simulink model "Copy_of_finalMG"  (R2025b)
settings: Solver=FixedStepAuto  StartTime=0.0  StopTime=.072  FixedStep=Ts  MaxStep=1e-4  RelTol=1e-3  EnableMultiTasking=on
PreLoadFcn:
  | Ts = 1e-5;
  | fsw = 1e3;
undefined symbols (not defined in the file or in its folder): localhost
libraries: nesl_utility x27, ee_lib x16, fl_lib x10, modbuslib x5, simulink x2, batteryecm_lib x1, eePwmGeneratorTwoLevel x1
CloseFcn:
  | try,close(h1_TwoLevelPWMGenerator),end
  | clear h1_TwoLevelPWMGenerator tout
  | 
  | clear simlog_TwoLevelPWMGenerator
  | clear logsout_TwoLevelPWMGenerator
  | clear Ts fsw
Description:
  | Three-Phase Two-Level PWM Generator
settings Model: Creator=The MathWorks, Inc.  LastModifiedBy=mattpenne
settings SolverCC: AlgebraicLoopSolver=TrustRegion  MaxZcPerStep=1.0
settings DataIOCC: LimitDataPoints=on  MaxDataPoints=50000  SaveFormat=Array  SaveOutput=off  SignalLogging=off  DSMLogging=off  SaveTime=off  ReturnWorkspaceOutputs=off  SignalLoggingName=logsout_TwoLevelPWMGenerator
settings OptimizationCC: ReuseModelBlockBuffer=off  LifeSpan=inf
settings DebuggingCC: AlgebraicLoopMsg=error  SolverPrmCheckMsg=warning  MultiTaskRateTransMsg=warning  UnconnectedInputMsg=warning  UnconnectedOutputMsg=warning  UnconnectedLineMsg=warning  AllowSymbolicDim=off  SFUnexpectedBacktrackingDiag=warning  SFNoUnconditionalDefaultTransitionDiag=warning  SFExecutionAtInitializationDiag=none  ArithmeticOperatorsInVariantConditions=warning
settings HardwareCC: ProdBitPerPointer=32.0  ProdBitPerSizeT=32.0  ProdBitPerPtrDiffT=32.0  ProdLargestAtomicFloat=None  ProdIntDivRoundTo=Undefined  ProdEndianess=Unspecified  ProdWordSize=32.0  ProdHWDeviceType=32-bit Generic
settings ModelReferenceCC: EnableRefExpFcnMdlSchedulingChecks=on  PropagateSignalLabelsOutOfModel=off
settings SFSimCC: SimUseLocalCustomCode=off  CustomCodeUndefinedFunction=UseInterfaceOnly
settings RTWCC: RTWUseLocalCustomCode=off  GPUComputeCapability=3.5  DLArmComputeVersion=19.05
settings CodeAppCC: StateflowObjectComments=on
settings GRTTargetCC: TargetLangStandard=C89/C90 (ANSI)
settings ConfigComp: CovMetricSettings=dw  CovSaveCumulativeToWorkspaceVar=on  CovSaveSingleToWorkspaceVar=on  CovExternalEMLEnable=off  CovSFcnEnable=off
settings SimscapeCC: SimscapeLogType=all  SimscapeLogSimulationStatistics=on  SimscapeLogName=simlog_TwoLevelPWMGenerator  SimscapeLogDataHistory=50000.0

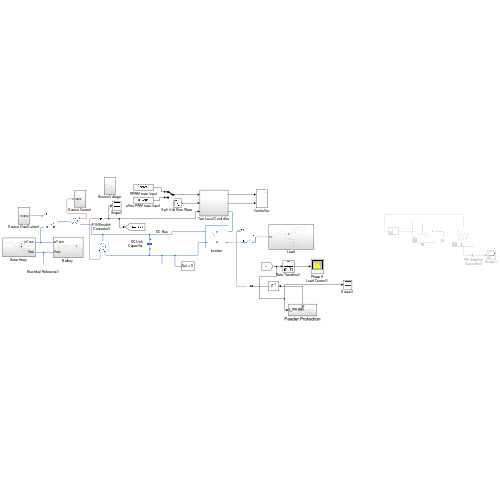
[thumbnail: Simulink's stored preview of the top-level diagram]
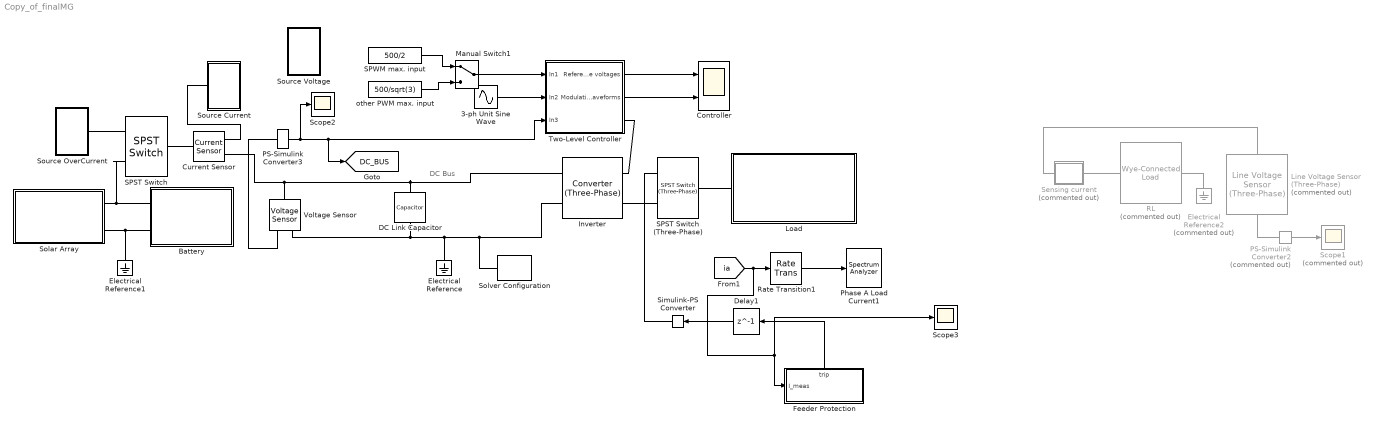
== system Copy_of_finalMG ==
  note: DC Bus
  3-ph Unit Sine Wave : Sin  Frequency=2*pi*60  Phase="[0  -2*pi/3  2*pi/3] + pi/2"  SampleTime=0
  Battery : Subsystem
  Controller : Scope  NumInputPorts=2
      settings: ActiveDisplayYMinimum=-250  ActiveDisplayYMaximum=250  DataLoggingVariableName=ScopeData2  DataLoggingSaveFormat=Array
  Current Sensor : fl_lib/Electrical/Electrical Sensors/Current Sensor
  DC Link Capacitor : ee_lib/Passive/Capacitor  cap_option=ee.enum.passive.capacitor.capOption.const  c=.001 F  Cvec=[1e-05, 1e-06] F  Vvec=[0, 10] V  CV_table_symmetry=ee.enum.passive.capacitor.tableSymmetry.yes  f_vec=[1, 10] kHz  DFext_vec=[.8, 1.2]  enable_C_tol=ee.enum.toleranceApplication.none  averaging_period=0 s  C_tol=5  tol_distribution=ee.enum.toleranceDistribution.uniform  nSigma=4  r=1e-6 Ohm  g=0 1/Ohm  enable_operating_limits=ee.enum.enable.no  operating_limit_action=ee.enum.passive.reportOpLim.warn  max_working_voltage_range=[-25, 25] V  power_rating=1 W  maxTemperature=85 degC  thermalEnable=false  thermalMass=1 J/K  i_specify=off  i_priority=None  i=0 A  i_nominal_specify=off  i_nominal_value=1  i_nominal_unit=A  v_specify=off  v_priority=None  v=0 V  v_nominal_specify=off  v_nominal_value=1  v_nominal_unit=V  vc_specify=off  vc_priority=High  vc=0 V  vc_nominal_specify=off  vc_nominal_value=1  vc_nominal_unit=V  T_specify=off  T_priority=None  T=298.15 K  T_nominal_specify=off  T_nominal_value=1  T_nominal_unit=K
  Delay1 : Delay  DelayLength=1  InitialCondition=0
  Electrical Reference : fl_lib/Electrical/Electrical Elements/Electrical Reference
  Electrical Reference1 : fl_lib/Electrical/Electrical Elements/Electrical Reference
  Electrical Reference2 : fl_lib/Electrical/Electrical Elements/Electrical Reference  Commented=on
  Feeder Protection : Subsystem
      settings: PortSchema="{\"entries\":[{\"content\":{\"sides\":[{\"content\":{\"connectorIds\":[\"In1\"]},\"type\":\"ConnectorPlacement.EquallySpacedRectSide\",\"uuid\":\"0697f356-98a9-46a1-9ee7-a2f5bd8a9ce9\"},{\"content\":{\"side\":\"RIGHT\"},\"type\":\"ConnectorPlacement.EquallySpacedRectSide\",\"uuid\":\"d4eac892-3d6d-4f1e-85a9-65422e23728d\"},{\"content\":{\"connectorIds\":[\"Out1\"],\"side\":\"TOP\"},\"type\":\"ConnectorPlacement.EquallySpacedRectSide\",\"uuid\":\"7d3e352e-ceac-4059-a935-aae4fffcf2cb\"}]},\"type\":\"ConnectorPlacement.EquallySpacedConnector\",\"uuid\":\"a2d9bf32-257e-4270-ae17-1068e4e35877\"}],\"packageUris\":[\"http://schema.mathworks.com/mf0/Connector/R2020b\"],\"version\":\"1.0\"}"
  Inverter : ee_lib/Semiconductors & Converters/Converters/Converter (Three-Phase)  port_option=ee.enum.threePhasePort.composite  fidelity_option=ee.enum.converters.fidelity.detailed  device_type=3  showThermalPort=false  K=0  Vth=0.5 V  Vgt=1 V  Vgt_off=-1 V  Ih=1 A  Vf=0.8 V  Ron=0.001 Ohm  Rds=0.001 Ohm  Goff=1e-5 1/Ohm  Eon_scalar=22.86e-3 J  Eoff_scalar=17.14e-3 J  Eoff_natural_commutation=10e-3 J  Voff=300 V  Iout_scalar=600 A  onCurrentMeasDelay=0 s  useCurrentFromPreviousCycle=false  useVoltageFromPreviousCycle=false  diode_param=2  diode_Vf=0.8 V  diode_Ron=0.001 Ohm  diode_Goff=1e-5 1/Ohm  diode_C=50 nF  diode_iRM=-235 A  diode_iF=300 A  diode_idot=-50 A/us  diode_trr_param=1  diode_trr_factor=3  diode_trr=15 us  diode_Qrr=1.5e+3 s*uA  diode_rec_loss_model=ee.enum.diode.reverseRecoveryModel.fixed  diode_ErecVal=0 J  diode_scaleWithIandV=false  diode_ErecMat=zeros(2, 3) J  diode_TjrecVec=[298.15, 398.15] K  diode_IfrecVec=[.1, 1, 10] A  diode_IrecVal=10 A  diode_VrecVal=10 V  diode_tFilter=1 / 1000 / 100 s  thermal_network_parameterization=ee.enum.thermalNetworkTopology.external  Rth=[.08, .5] K/W  Rth_Cauer=[.08, .1, .5] K/W  Rth_Foster=[.08, .14, .22, .16] K/W  thermal_mass_parameterization=ee.enum.thermalNetwork.timeconstant  thermal_mass=[.01, .5] J/K  thermal_mass_Cauer=[.01, .1, .5] J/K  thermal_mass_Foster=[.001, .005, .05, .5] J/K  thermal_time_constant=[.001, .2] s  thermal_time_constant_Cauer=[.001, .1, .2] s  thermal_time_constant_Foster=[7e-05, .0007, .01, .08] s  thermal_mass_initial_temperatures=[25, 25] degC  thermal_mass_initial_temperatures_Cauer=[25, 25, 25] degC  junction_thermal_mass=0.01 J/K  Tvec_initial_Foster=[25, 25, 25, 25] degC  snubber_type=0  Cs=1e-7 F  Rs=0.1 Ohm  Vce_loss=[0, 150, 300] V
  Line Voltage Sensor (Three-Phase) : ee_lib/Sensors & Transducers/Line Voltage Sensor (Three-Phase)  Commented=on
  Load : Subsystem
  Manual Switch1 : ManualSwitch
  PS-Simulink Converter2 : nesl_utility/PS-Simulink Converter  Commented=on  PhysicalDomain=network_engine_domain  SubClassName=ps_output  LeftPortType=input  RightPortType=output  PseudoPeriodic=off  Frequencies=[]  VectorFormat=inherit  Unit=inherit  AffineConversion=off
  PS-Simulink Converter3 : nesl_utility/PS-Simulink Converter  PhysicalDomain=network_engine_domain  SubClassName=ps_output  LeftPortType=input  RightPortType=output  PseudoPeriodic=off  Frequencies=[]  VectorFormat=inherit  Unit=inherit  AffineConversion=off
  Phase A Load Current1 : SpectrumAnalyzer  WindowPosition=[135.000000,120.000000,1010.000000,481.000000,]  ScopeFrameLocation=window  SpectrumType=RMS  Method=Welch  PlotAsTwoSidedSpectrum=off  AxesScaling=Manual  RBWSource=Property  RBW=9  Span=5000  CenterFrequency=2500  StartFrequency=0  OverlapPercent=90  AveragingMethod=Running  SpectrumUnits=Vrms  YLimits=[-6.549396466439435 13.341492111050359]  SelectedToolstripTab=spectrumAnalyzerToolstrip.channelMeasurementsTab  AllowFFTLengthLessThanSamplesPerUpdate=on
  RL : ee_lib/Passive/RLC Assemblies/Wye-Connected Load  Commented=on  port_option=ee.enum.threePhasePort.composite  parameterization=1  component_structure=4  component_structure_PQ=1  R=100 Ohm  L=0.001 H  C=1e-6 F  VRated=2.4e+4 V  FRated=60 Hz  P=1000 W  Qpos=100 V*A  Qneg=-100 V*A  R_parasitic=1e-6 Ohm  G_parasitic=1e-6 1/Ohm  R_parasitic_PQ=1e-6 Ohm  G_parasitic_PQ=1e-6 1/Ohm  Vmag0=2.4e+4 V  Vang0=0 deg  Freq0=60 Hz  IL_specify=on  IL_priority=High  IL=[ 0 0 0 ] A  IL_nominal_specify=off  IL_nominal_value=1  IL_nominal_unit=A  VC_specify=on  VC_priority=High  VC=[ 0 0 0 ] V  VC_nominal_specify=off  VC_nominal_value=1  VC_nominal_unit=V
  Rate Transition1 : RateTransition  OutPortSampleTime=1e-4
  SPST Switch : ee_lib/Switches & Breakers/SPST Switch  R_closed=0.01 Ohm  G_open=1e-6 S  Threshold=0.5 V  Width=0 V  model_dynamics=0  t_on=1e-3 s  t_off=1e-3 s  initial_vT=0 V
      settings: InternalSimscapePortConfiguration="{\"Bottom\":[],\"Left\":[{\"id\":\"vT\",\"label\":\"vT\",\"type\":\"input\"},{\"id\":\"p\",\"label\":\"\",\"type\":\"foundation.electrical.electrical\"}],\"Right\":[{\"id\":\"n\",\"label\":\"\",\"type\":\"foundation.electrical.electrical\"}],\"Top\":[]}"
  SPST Switch (Three-Phase) : ee_lib/Switches & Breakers/SPST Switch (Three-Phase)  R_closed=0.001 Ohm  G_open=1e-6 1/Ohm  threshold=0.5 V  i_vT_specify=off  i_vT_priority=None  i_vT=0 A  i_vT_nominal_specify=off  i_vT_nominal_value=1  i_vT_nominal_unit=A  I_specify=off  I_priority=None  I=[0, 0, 0] A  I_nominal_specify=off  I_nominal_value=1  I_nominal_unit=A  V_specify=off  V_priority=None  V=[0, 0, 0] V  V_nominal_specify=off  V_nominal_value=1  V_nominal_unit=V  i_a_specify=off  i_a_priority=None  i_a=0 A  i_a_nominal_specify=off  i_a_nominal_value=1  i_a_nominal_unit=A  v_a_specify=off  v_a_priority=None  v_a=0 V  v_a_nominal_specify=off  v_a_nominal_value=1  v_a_nominal_unit=V  i_b_specify=off  i_b_priority=None  i_b=0 A  i_b_nominal_specify=off  i_b_nominal_value=1  i_b_nominal_unit=A  v_b_specify=off  v_b_priority=None  v_b=0 V  v_b_nominal_specify=off  v_b_nominal_value=1  v_b_nominal_unit=V  i_c_specify=off  i_c_priority=None  i_c=0 A  i_c_nominal_specify=off  i_c_nominal_value=1  i_c_nominal_unit=A  v_c_specify=off  v_c_priority=None  v_c=0 V  v_c_nominal_specify=off  v_c_nominal_value=1  v_c_nominal_unit=V
      settings: InternalSimscapePortConfiguration="{\"Bottom\":[],\"Left\":[{\"id\":\"vT\",\"label\":\"vT\",\"type\":\"input\"},{\"id\":\"N1\",\"label\":\"~1\",\"type\":\"foundation.electrical.three_phase\"}],\"Right\":[{\"id\":\"N2\",\"label\":\"~2\",\"type\":\"foundation.electrical.three_phase\"}],\"Top\":[]}"
  SPWM max. input : Constant  Value=500/2
  Scope1 : Scope  Commented=on
      settings: ActiveDisplayYMinimum=-1.3412361067423506  ActiveDisplayYMaximum=1.8250988567194808
  Scope2 : Scope
      settings: ActiveDisplayYMinimum=-157.006255276564  ActiveDisplayYMaximum=731.00271353862377  DataLoggingVariableName=ScopeData2
  Scope3 : Scope
      settings: ActiveDisplayYMinimum=-3.9834223121719612  ActiveDisplayYMaximum=2.6570930010278939
  Sensing current : Subsystem  Commented=on
      mask Display: disp('i')
  Simulink-PS Converter : nesl_utility/Simulink-PS Converter  PhysicalDomain=network_engine_domain  SubClassName=ps_input  LeftPortType=input  RightPortType=output  PseudoPeriodic=off  Frequencies=[]  NoiseDistribution=none  NoiseParameters=[]  Unit=1  AffineConversion=off  FilteringAndDerivatives=provide  SimscapeFilterOrder=1  InputFilterTimeConstant=0.001  UdotUserProvided=0
  Solar Array : Subsystem
  Solver Configuration : nesl_utility/Solver Configuration  PhysicalDomain=network_engine_domain  SubClassName=solver  LeftPortType=input  RightPortType=generic  Tones=[]  Harmonics=[]  SimulateNoise=off  Profile=off  UseLocalSampling=off  EnableSwitchedLinearOptims=on  FrequencyDomain=off  UseCCode=off  RelTol=0.001  AbsTol=1e-06  MinStep=1e-09  ToWorkspace=off  RevertToSquareIcSolve=off  NumHomotopyIterations=100  PhasorMode=off  PhasorModeNumHarmonics=1  ConsistencySolver=NEWTON_FTOL  IndexReductionMethod=DerivativeReplacement  DoDC=off  ResidualTolerance=1e-09  ConsistencyTolSource=GLOBAL  ConsistencyAbsTol=0.001  ConsistencyRelTol=0.001  ConsistencyTolFactor=0.001  UseLocalSolver=on  LocalSolverChoice=NE_BACKWARD_EULER_ADVANCER  ResolveIndetEquations=on  FunctionEvalNumThread=1  LocalSolverSampleTime=0.0001  DoFixedCost=off  MaxNonlinIter=3  MaxModeIter=2  ComputeImpulses=off  ImpulseIterations=2  LinearAlgebra=auto  LinearAlgebraNumThread=0  EquationFormulation=NE_TIME_EF  DelaysMemoryBudget=1024  AutomaticFiltering=on  FilteringTimeConstant=0.001  PartitionStorageMethod=AS_NEEDED  PartitionMemoryBudget=1024  PartitionMethod=FAST  MultibodyUseLocalSolver=off  MultibodyLocalSolverChoice=ODE1  MultibodyLocalSolverSampleTime=0.001
  Source Current : Subsystem
  Source OverCurrent : Subsystem
  Source Voltage : Subsystem
  Two-Level Controller : Subsystem
  Voltage Sensor : fl_lib/Electrical/Electrical Sensors/Voltage Sensor
  other PWM max. input : Constant  Value=500/sqrt(3)
  tag scope: DC_BUS=global
  wires:
  other PWM max. input/1 -> Manual Switch1/2
  SPWM max. input/1 -> Manual Switch1/1
  Manual Switch1/1 -> Two-Level Controller/1(In1)
  3-ph Unit Sine Wave/1 -> Two-Level Controller/2(In2)
  PS-Simulink Converter3/1 -> Scope2/1, [DC_BUS], Two-Level Controller/3(In3)
  Two-Level Controller/1(Reference voltages) -> Controller/1
  Two-Level Controller/2(Modulation waveforms) -> Controller/2
  PS-Simulink Converter2/1 -> Scope1/1
  Rate Transition1/1 -> Phase A Load Current1/1
  Feeder Protection/1(trip) -> Delay1/1
  Delay1/1 -> Simulink-PS Converter/1
  [ia] -> Scope3/1, Feeder Protection/1(I_meas), Rate Transition1/1
  connections:
  RL/RConn1 -- Electrical Reference2/LConn1
  Line Voltage Sensor (Three-Phase)/LConn1 -- Sensing current/LConn1
  Two-Level Controller/RConn1 -- Inverter/LConn1
  PS-Simulink Converter2/LConn1 -- Line Voltage Sensor (Three-Phase)/RConn1
  Battery/LConn2 -- Solar Array/RConn2 -- Electrical Reference1/LConn1
  Voltage Sensor/RConn1 -- PS-Simulink Converter3/LConn1
  Electrical Reference/LConn1 -- Solver Configuration/RConn1 -- Inverter/RConn2 -- Voltage Sensor/RConn2 -- DC Link Capacitor/RConn1
  Battery/LConn1 -- SPST Switch/LConn2 -- Solar Array/RConn1
  Sensing current/RConn1 -- RL/LConn1
  SPST Switch (Three-Phase)/LConn2 -- Inverter/LConn2
  Simulink-PS Converter/RConn1 -- SPST Switch (Three-Phase)/LConn1
  Source OverCurrent/RConn1 -- SPST Switch/LConn1
  Source Current/LConn1 -- Current Sensor/RConn1
  DC Link Capacitor/LConn1 -- Current Sensor/RConn2 -- Voltage Sensor/LConn1 -- Inverter/RConn1
  Current Sensor/LConn1 -- SPST Switch/RConn1
  Load/LConn1 -- SPST Switch (Three-Phase)/RConn1

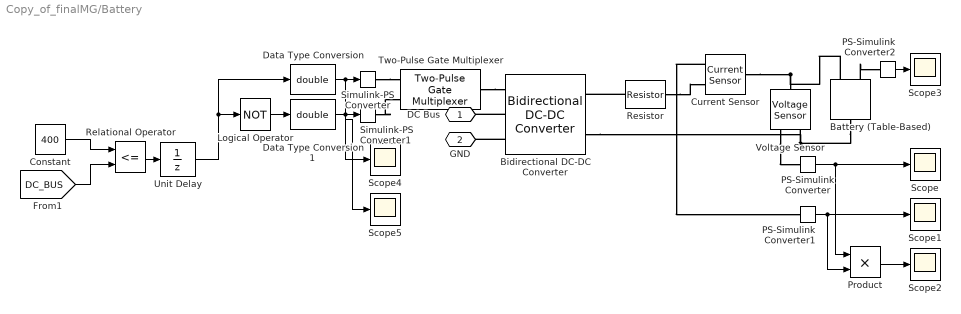
== system Copy_of_finalMG/Battery ==
  Battery (Table-Based) : batteryecm_lib/Battery (Table-Based)  SOC_vec=[0, .1, .25, .5, .75, .9, 1]  T_dependence=simscape.enum.tablebattery.temperature_dependence.yes  prm_dir=simscape.enum.tablebattery.prm_dir.noCurrentDirectionality  T_vec=[278, 293, 313] K  V0_mat=|  V0_vec=[3.5057, 3.566, 3.6337, 3.7127, 3.9259, 4.0777, 4.1928] V  V_range=[0, inf] V  R0_mat=[.0117, .0085, .009; .011, .0085, .009; .0114, .0087, .0092; .0107, .0082, .0088; .0107, .0083, .0091; .0113, .0085, .0089; .0116, .0085, .0089] Ohm  R0_vec=[.0085, .0085, .0087, .0082, .0083, .0085, .0085] Ohm  R0_dis_mat=[.0117, .0085, .009; .011, .0085, .009; .0114, .0087, .0092; .0107, .0082, .0088; .0107, .0083, .0091; .0113, .0085, .0089; .0116, .0085, .0089] Ohm  R0_dis_vec=[.0085, .0085, .0087, .0082, .0083, .0085, .0085] Ohm  R0_ch_mat=[.0117, .0085, .009; .011, .0085, .009; .0114, .0087, .0092; .0107, .0082, .0088; .0107, .0083, .0091; .0113, .0085, .0089; .0116, .0085, .0089] Ohm  R0_ch_vec=[.0085, .0085, .0087, .0082, .0083, .0085, .0085] Ohm  AH=2700 A*hr  prm_leak=simscape.enum.tablebattery.prm_leak.disabled  Rleak_vec=[8000, 7000, 6000] Ohm  Rleak=7e3 Ohm  extrapolation_option=simscape.enum.extrapolation.nearest  SOC_port=simscape.enum.tablebattery.enable.yes  prm_dyn=simscape.enum.tablebattery.prm_dyn.off  R1_mat=[.0109, .0029, .0013; .0069, .0024, .0012; .0047, .0026, .0013; .0034, .0016, .001; .0033, .0023, .0014; .0033, .0018, .0011; .0028, .0017, .0011] Ohm  R1_vec=[.0029, .0024, .0026, .0016, .0023, .0018, .0017] Ohm  tau1_mat=[20, 36, 39; 31, 45, 39; 109, 105, 61; 36, 29, 26; 59, 77, 67; 40, 33, 29; 25, 39, 33] s  tau1_vec=[36, 45, 105, 29, 77, 33, 39] s  R2_mat=[.0109, .0029, .0013; .0069, .0024, .0012; .0047, .0026, .0013; .0034, .0016, .001; .0033, .0023, .0014; .0033, .0018, .0011; .0028, .0017, .0011] Ohm  R2_vec=[.0029, .0024, .0026, .0016, .0023, .0018, .0017] Ohm  tau2_mat=[20, 36, 39; 31, 45, 39; 109, 105, 61; 36, 29, 26; 59, 77, 67; 40, 33, 29; 25, 39, 33] s  tau2_vec=[36, 45, 105, 29, 77, 33, 39] s  R3_mat=[.0109, .0029, .0013; .0069, .0024, .0012; .0047, .0026, .0013; .0034, .0016, .001; .0033, .0023, .0014; .0033, .0018, .0011; .0028, .0017, .0011] Ohm  R3_vec=[.0029, .0024, .0026, .0016, .0023, .0018, .0017] Ohm  tau3_mat=[20, 36, 39; 31, 45, 39; 109, 105, 61; 36, 29, 26; 59, 77, 67; 40, 33, 29; 25, 39, 33] s  tau3_vec=[36, 45, 105, 29, 77, 33, 39] s  R4_mat=[.0109, .0029, .0013; .0069, .0024, .0012; .0047, .0026, .0013; .0034, .0016, .001; .0033, .0023, .0014; .0033, .0018, .0011; .0028, .0017, .0011] Ohm  R4_vec=[.0029, .0024, .0026, .0016, .0023, .0018, .0017] Ohm  tau4_mat=[20, 36, 39; 31, 45, 39; 109, 105, 61; 36, 29, 26; 59, 77, 67; 40, 33, 29; 25, 39, 33] s  tau4_vec=[36, 45, 105, 29, 77, 33, 39] s  R5_mat=[.0109, .0029, .0013; .0069, .0024, .0012; .0047, .0026, .0013; .0034, .0016, .001; .0033, .0023, .0014; .0033, .0018, .0011; .0028, .0017, .0011] Ohm  R5_vec=[.0029, .0024, .0026, .0016, .0023, .0018, .0017] Ohm  tau5_mat=[20, 36, 39; 31, 45, 39; 109, 105, 61; 36, 29, 26; 59, 77, 67; 40, 33, 29; 25, 39, 33] s  tau5_vec=[36, 45, 105, 29, 77, 33, 39] s  prm_fade=simscape.enum.tablebattery.prm_fade.disabled  N0=100  dV0=0  dR0=0  dAH=0  dRleak=0  dR1=0  dR2=0  dR3=0  dR4=0  dR5=0  N0vec=[0, 100, 200, 300]  Tfadevec=[298.15, 323.15] K  dV0vec=[0, 0, 0, 0]  dR0vec=[0, 0, 0, 0]  dAHvec=[0, 0, 0, 0]  dRleakvec=[0, 0, 0, 0]  dR1vec=[0, 0, 0, 0]  dR2vec=[0, 0, 0, 0]  dR3vec=[0, 0, 0, 0]  dR4vec=[0, 0, 0, 0]  dR5vec=[0, 0, 0, 0]  dV0mat=[0, 0; 0, 0; 0, 0; 0, 0]  dR0mat=[0, 0; 0, 0; 0, 0; 0, 0]  dAHmat=[0, 0; 0, 0; 0, 0; 0, 0]  dRleakmat=[0, 0; 0, 0; 0, 0; 0, 0]  dR1mat=[0, 0; 0, 0; 0, 0; 0, 0]  dR2mat=[0, 0; 0, 0; 0, 0; 0, 0]  dR3mat=[0, 0; 0, 0; 0, 0; 0, 0]  dR4mat=[0, 0; 0, 0; 0, 0; 0, 0]  dR5mat=[0, 0; 0, 0; 0, 0; 0, 0]  prm_age_modeling=simscape.enum.tablebattery.prm_age_modeling.equation  storage_dt_age_vec=[0] d  storage_T_age_vec=[273] K  prm_age_OCV=simscape.enum.tablebattery.prm_age_OCV.OCV  OCV_age=0.9  SOC_age=0.6  prm_age_resistance=simscape.enum.tablebattery.prm_age.disabled  OCV_scaling_age_resistance=2.2134e6  OCV_offset_age_resistance=1.632e6  temp_exp_age_resistance=0.515833569 V  t_exp_age_resistance=0.75  T_age_vec_resistance=[273.15, 298.15, 323.15] K  dt_age_vec_resistance=[0, 90, 180, 270] d  dR0_age_vec=[0, 0, 0]  t_meas_dR0_age=100 d  dR0_age_mat=[0, 0, 0; 0, 0, 0; 0, 0, 0; 0, 0, 0]  prm_age_capacity=simscape.enum.tablebattery.prm_age.disabled  OCV_scaling_age_capacity=1.5097e07  OCV_offset_age_capacity=8.3625e06  temp_exp_age_capacity=0.6011 V  t_exp_age_capacity=0.75  T_age_vec_capacity=[273.15, 298.15, 323.15] K  dt_age_vec_capacity=[0, 90, 180, 270] d  dAH_age_vec=[0, 0, 0]  t_meas_dAH_age=100 d  dAH_age_mat=[0, 0, 0; 0, 0, 0; 0, 0, 0; 0, 0, 0]  thermal_port=simscape.enum.thermaleffects.omit  temperature=298.15 K  thermal_mass=100 J/K  i_specify=off  i_priority=None  i=0 A  i_nominal_specify=off  i_nominal_value=1  i_nominal_unit=A  v_specify=on  v_priority=Low  v=400 V  v_nominal_specify=off  v_nominal_value=1  v_nominal_unit=V  stateOfCharge_specify=on  stateOfCharge_priority=High  stateOfCharge=.5  stateOfCharge_nominal_specify=off  stateOfCharge_nominal_value=1  stateOfCharge_nominal_unit=1  num_cycles_specify=off  num_cycles_priority=High  num_cycles=0  num_cycles_nominal_specify=off  num_cycles_nominal_value=1  num_cycles_nominal_unit=1  cell_temperature_specify=off  cell_temperature_priority=High  cell_temperature=298.15 K  cell_temperature_nominal_specify=off  cell_temperature_nominal_value=1  cell_temperature_nominal_unit=K
      | [3490, 3500, 3510;
      |  3550, 3570, 3560;
      |  3620, 3630, 3640;
      |  3710, 3710, 3720;
      |  3910, 3930, 3940;
      |  4070, 4080, 4080;
      |  4190, 4190, 4190] V
      settings: InternalSimscapePortConfiguration="{\"Bottom\":[],\"Left\":[{\"id\":\"p\",\"label\":\"+\",\"type\":\"foundation.electrical.electrical\"},{\"id\":\"soc\",\"label\":\"SOC\",\"type\":\"output\"}],\"Right\":[{\"id\":\"n\",\"label\":\"-\",\"type\":\"foundation.electrical.electrical\"}],\"Top\":[]}"
  Bidirectional DC-DC Converter : ee_lib/Semiconductors & Converters/Converters/Bidirectional DC-DC Converter  fidelity_option=ee.enum.converters.fidelity.detailed  device_type=ee.enum.converters.switchingdevice.averaged  Vf=0.8 V  Ron=0.001 Ohm  Rds=0.001 Ohm  Goff=1e-5 1/Ohm  Vth=6 V  Vgt=1 V  Vgt_off=-1 V  Ih=1 A  K=0  diode_param=ee.enum.converters.diode.nodynamics  diode_Vf=0.8 V  diode_Ron=0.001 Ohm  diode_Goff=1e-5 1/Ohm  diode_C=50 nF  diode_iRM=-235 A  diode_iF=300 A  diode_idot=-50 A/us  diode_trr_param=ee.enum.converters.diodetrr.trr_factor  diode_trr_factor=3  diode_trr=15 us  diode_Qrr=1500 s*uA  L=1e-6 H  Rl=0 Ohm  C1=1e-7 F  C2=1e-7 F  R1=1e-6 Ohm  R2=1e-6 Ohm  snubber_type=ee.enum.converters.snubber.exclude  Cs=1e-7 F  Rs=0.1 Ohm  iL_specify=off  iL_priority=High  iL=0 A  iL_nominal_specify=off  iL_nominal_value=1  iL_nominal_unit=A  vc1_specify=off  vc1_priority=High  vc1=0 V  vc1_nominal_specify=off  vc1_nominal_value=1  vc1_nominal_unit=V  vc2_specify=off  vc2_priority=High  vc2=0 V  vc2_nominal_specify=off  vc2_nominal_value=1  vc2_nominal_unit=V  device_type_hv=ee.enum.converters.switchingdevice.ideal  Vf_hv=0.8 V  Ron_hv=0.001 Ohm  Rds_hv=0.001 Ohm  Goff_hv=1e-5 1/Ohm  Vth_hv=6 V  Vgt_hv=1 V  Vgt_off_hv=-1 V  Ih_hv=1 A  device_type_lv=ee.enum.converters.switchingdevice.ideal  Vf_lv=0.8 V  Ron_lv=0.001 Ohm  Rds_lv=0.001 Ohm  Goff_lv=1e-5 1/Ohm  Vth_lv=6 V  Vgt_lv=1 V  Vgt_off_lv=-1 V  Ih_lv=1 A  T_L1=0.03 H  T_L2=0.03 H  T_k=0.9  snubber_type_hv=ee.enum.converters.snubber.exclude  Cs_hv=1e-7 F  Rs_hv=0.1 Ohm  snubber_type_lv=ee.enum.converters.snubber.exclude  Cs_lv=1e-7 F  Rs_lv=0.1 Ohm  iL1_specify=off  iL1_priority=High  iL1=0 A  iL1_nominal_specify=off  iL1_nominal_value=1  iL1_nominal_unit=A  iL2_specify=off  iL2_priority=High  iL2=0 A  iL2_nominal_specify=off  iL2_nominal_value=1  iL2_nominal_unit=A  hysteresisCurrent=0.0005 A
      settings: InternalSimscapePortConfiguration="{\"Bottom\":[],\"Left\":[{\"id\":\"G\",\"label\":\"G\",\"type\":\"foundation.electrical.four_phase\"},{\"id\":\"p1\",\"label\":\"1+\",\"type\":\"foundation.electrical.electrical\"},{\"id\":\"n1\",\"label\":\"1-\",\"type\":\"foundation.electrical.electrical\"}],\"Right\":[{\"id\":\"p2\",\"label\":\"2+\",\"type\":\"foundation.electrical.electrical\"},{\"id\":\"n2\",\"label\":\"2-\",\"type\":\"foundation.electrical.electrical\"}],\"Top\":[]}"
  Constant : Constant  Value=400
  Current Sensor : fl_lib/Electrical/Electrical Sensors/Current Sensor
  Data Type Conversion : DataTypeConversion  OutDataTypeStr=double  SaturateOnIntegerOverflow=off  RndMeth=Floor
  Data Type Conversion1 : DataTypeConversion  OutDataTypeStr=double  SaturateOnIntegerOverflow=off  RndMeth=Floor
  Logical Operator : Logic  Operator=NOT  AllPortsSameDT=off  OutDataTypeStr=boolean
  PS-Simulink Converter : nesl_utility/PS-Simulink Converter  PhysicalDomain=network_engine_domain  SubClassName=ps_output  LeftPortType=input  RightPortType=output  PseudoPeriodic=off  Frequencies=[]  VectorFormat=inherit  Unit=inherit  AffineConversion=off
  PS-Simulink Converter1 : nesl_utility/PS-Simulink Converter  PhysicalDomain=network_engine_domain  SubClassName=ps_output  LeftPortType=input  RightPortType=output  PseudoPeriodic=off  Frequencies=[]  VectorFormat=inherit  Unit=inherit  AffineConversion=off
  PS-Simulink Converter2 : nesl_utility/PS-Simulink Converter  PhysicalDomain=network_engine_domain  SubClassName=ps_output  LeftPortType=input  RightPortType=output  PseudoPeriodic=off  Frequencies=[]  VectorFormat=inherit  Unit=inherit  AffineConversion=off
  Product : Product
  Relational Operator : RelationalOperator  Operator=<=  OutDataTypeStr=boolean  RndMeth=Simplest  InputSameDT=off
  Resistor : fl_lib/Electrical/Electrical Elements/Resistor  R=5 Ohm  i_specify=off  i_priority=None  i=0 A  i_nominal_specify=off  i_nominal_value=1  i_nominal_unit=A  v_specify=off  v_priority=None  v=0 V  v_nominal_specify=off  v_nominal_value=1  v_nominal_unit=V
  Scope{,1..5} (6 alike) : Scope
      Scope settings: ActiveDisplayYMinimum=3712.522737924663  ActiveDisplayYMaximum=3712.6272619797123  DataLoggingVariableName=ScopeData2
      Scope1 settings: ActiveDisplayYMinimum=-6.25  ActiveDisplayYMaximum=6.25  DataLoggingVariableName=ScopeData3
      Scope2 settings: ActiveDisplayYMinimum=-1  ActiveDisplayYMaximum=1  DataLoggingVariableName=ScopeData4
      Scope3 settings: ActiveDisplayYMinimum=-1  ActiveDisplayYMaximum=1  DataLoggingVariableName=ScopeData6
      Scope4 settings: ActiveDisplayYMinimum=-1  ActiveDisplayYMaximum=1  DataLoggingVariableName=ScopeData7
      Scope5 settings: ActiveDisplayYMinimum=-1  ActiveDisplayYMaximum=1  DataLoggingVariableName=ScopeData8
  Simulink-PS Converter : nesl_utility/Simulink-PS Converter  PhysicalDomain=network_engine_domain  SubClassName=ps_input  LeftPortType=input  RightPortType=output  PseudoPeriodic=off  Frequencies=[]  NoiseDistribution=none  NoiseParameters=[]  Unit=1  AffineConversion=off  FilteringAndDerivatives=provide  SimscapeFilterOrder=1  InputFilterTimeConstant=0.001  UdotUserProvided=0
  Simulink-PS Converter1 : nesl_utility/Simulink-PS Converter  PhysicalDomain=network_engine_domain  SubClassName=ps_input  LeftPortType=input  RightPortType=output  PseudoPeriodic=off  Frequencies=[]  NoiseDistribution=none  NoiseParameters=[]  Unit=1  AffineConversion=off  FilteringAndDerivatives=provide  SimscapeFilterOrder=1  InputFilterTimeConstant=0.001  UdotUserProvided=0
  Two-Pulse Gate Multiplexer : ee_lib/Semiconductors & Converters/Converters/Two-Pulse Gate Multiplexer  port_option=ee.enum.controlport.ps
      settings: InternalSimscapePortConfiguration="{\"Bottom\":[],\"Left\":[{\"id\":\"G1_ps\",\"label\":\"G1\",\"type\":\"input\"},{\"id\":\"G2_ps\",\"label\":\"G2\",\"type\":\"input\"}],\"Right\":[{\"id\":\"p\",\"label\":\"G\",\"type\":\"foundation.electrical.four_phase\"}],\"Top\":[]}"
  Unit Delay : UnitDelay  SampleTime=-1  HasFrameUpgradeWarning=on
  Voltage Sensor : fl_lib/Electrical/Electrical Sensors/Voltage Sensor
  DC Bus : PMIOPort  Side=Left
  GND : PMIOPort  Port=2  Side=Left
  wires:
  PS-Simulink Converter/1 -> Product/1, Scope/1
  Product/1 -> Scope2/1
  PS-Simulink Converter1/1 -> Scope1/1, Product/2
  PS-Simulink Converter2/1 -> Scope3/1
  [DC_BUS] -> Relational Operator/2
  Data Type Conversion1/1 -> Scope5/1, Simulink-PS Converter1/1
  Relational Operator/1 -> Unit Delay/1
  Unit Delay/1 -> Logical Operator/1, Data Type Conversion/1
  Data Type Conversion/1 -> Scope4/1, Simulink-PS Converter/1
  Logical Operator/1 -> Data Type Conversion1/1
  Constant/1 -> Relational Operator/1
  connections:
  Bidirectional DC-DC Converter/LConn3 -- GND/RConn1
  Battery (Table-Based)/LConn2 -- PS-Simulink Converter2/LConn1
  Bidirectional DC-DC Converter/LConn2 -- DC Bus/RConn1
  Battery (Table-Based)/LConn1 -- Current Sensor/LConn1 -- Voltage Sensor/LConn1
  Battery (Table-Based)/RConn1 -- Bidirectional DC-DC Converter/RConn2 -- Voltage Sensor/RConn2
  Two-Pulse Gate Multiplexer/RConn1 -- Bidirectional DC-DC Converter/LConn1
  Simulink-PS Converter1/RConn1 -- Two-Pulse Gate Multiplexer/LConn2
  Simulink-PS Converter/RConn1 -- Two-Pulse Gate Multiplexer/LConn1
  Voltage Sensor/RConn1 -- PS-Simulink Converter/LConn1
  Current Sensor/RConn1 -- PS-Simulink Converter1/LConn1
  Resistor/LConn1 -- Bidirectional DC-DC Converter/RConn1
  Resistor/RConn1 -- Current Sensor/RConn2

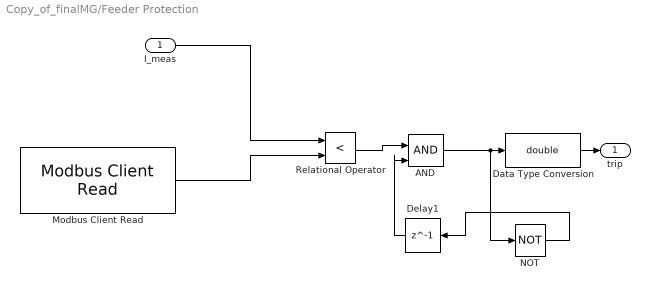
== system Copy_of_finalMG/Feeder Protection ==
  I_meas : Inport
  AND : Logic  IconShape=distinctive  AllPortsSameDT=off  OutDataTypeStr=boolean
  Data Type Conversion : DataTypeConversion  OutDataTypeStr=double  SaturateOnIntegerOverflow=off  RndMeth=Floor
  Delay1 : Delay  DelayLength=1  InitialCondition=0
  Modbus Client Read : modbuslib/Modbus Client Read  RetainClient=ModbusClient  ClientList=ModbusClient  ConnectionEndpoint=localhost:502  ServerId=1  RegisterTable={ '1', 'I_comm', '3', 'Holding Register', 'double', '1' }  SampleTime=-1
  NOT : Logic  Operator=NOT  IconShape=distinctive  AllPortsSameDT=off  OutDataTypeStr=boolean
  Relational Operator : RelationalOperator  Operator=<  OutDataTypeStr=boolean  RndMeth=Simplest  InputSameDT=off
  trip : Outport
  wires:
  Modbus Client Read/1 -> Relational Operator/2
  I_meas/1 -> Relational Operator/1
  Relational Operator/1 -> AND/1
  Data Type Conversion/1 -> trip/1
  Delay1/1 -> AND/2
  AND/1 -> NOT/1, Data Type Conversion/1
  NOT/1 -> Delay1/1

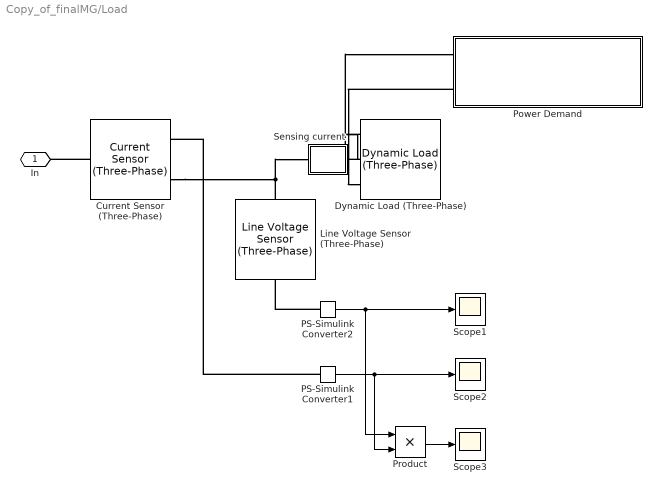
== system Copy_of_finalMG/Load ==
  Current Sensor (Three-Phase) : ee_lib/Sensors & Transducers/Current Sensor (Three-Phase)
  Dynamic Load (Three-Phase) : ee_lib/Passive/Dynamic Load (Three-Phase)  port_option=ee.enum.threePhasePort.composite  FRated=60 Hz  Vline_rms_min=10 V  tau=0.01 s  Vline_rms_ini=10 V  Vang_ini=0 deg  gmin=0 S
      settings: InternalSimscapePortConfiguration="{\"Bottom\":[],\"Left\":[{\"id\":\"N\",\"label\":\"~\",\"type\":\"foundation.electrical.three_phase\"}],\"Right\":[],\"Top\":[{\"id\":\"P\",\"label\":\"P\",\"type\":\"input\"},{\"id\":\"Q\",\"label\":\"Q\",\"type\":\"input\"}]}"
  Line Voltage Sensor (Three-Phase) : ee_lib/Sensors & Transducers/Line Voltage Sensor (Three-Phase)
  PS-Simulink Converter1 : nesl_utility/PS-Simulink Converter  PhysicalDomain=network_engine_domain  SubClassName=ps_output  LeftPortType=input  RightPortType=output  PseudoPeriodic=off  Frequencies=[]  VectorFormat=inherit  Unit=inherit  AffineConversion=off
  PS-Simulink Converter2 : nesl_utility/PS-Simulink Converter  PhysicalDomain=network_engine_domain  SubClassName=ps_output  LeftPortType=input  RightPortType=output  PseudoPeriodic=off  Frequencies=[]  VectorFormat=inherit  Unit=inherit  AffineConversion=off
  Power Demand : Subsystem
  Product : Product
  Scope1 : Scope
      settings: ActiveDisplayYMinimum=-2.5359903368699639  ActiveDisplayYMaximum=3.7660193798932835
  Scope2 : Scope
      settings: ActiveDisplayYMinimum=-57.921103589266146  ActiveDisplayYMaximum=61.173869519283421  DataLoggingVariableName=ScopeData10
  Scope3 : Scope
      settings: ActiveDisplayYMinimum=-145.06724335949744  ActiveDisplayYMaximum=161.387603824085  DataLoggingVariableName=ScopeData11
  Sensing current : Subsystem
      mask Display: disp('i')
  In : PMIOPort  Side=Left
  wires:
  PS-Simulink Converter2/1 -> Product/1, Scope1/1
  PS-Simulink Converter1/1 -> Product/2, Scope2/1
  Product/1 -> Scope3/1
  connections:
  Dynamic Load (Three-Phase)/LConn1 -- Sensing current/RConn1
  Power Demand/LConn2 -- Dynamic Load (Three-Phase)/LConn3
  Dynamic Load (Three-Phase)/LConn2 -- Power Demand/LConn1
  PS-Simulink Converter2/LConn1 -- Line Voltage Sensor (Three-Phase)/RConn1
  Line Voltage Sensor (Three-Phase)/LConn1 -- Sensing current/LConn1 -- Current Sensor (Three-Phase)/RConn2
  Current Sensor (Three-Phase)/LConn1 -- In/RConn1
  PS-Simulink Converter1/LConn1 -- Current Sensor (Three-Phase)/RConn1

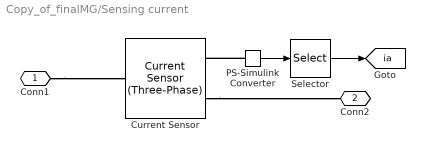
== system Copy_of_finalMG/Sensing current ==
  Current Sensor : ee_lib/Sensors & Transducers/Current Sensor (Three-Phase)
  PS-Simulink Converter : nesl_utility/PS-Simulink Converter  PhysicalDomain=network_engine_domain  SubClassName=ps_output  LeftPortType=input  RightPortType=output  PseudoPeriodic=off  Frequencies=[]  VectorFormat=1-D array  Unit=1  AffineConversion=off
  Selector : Selector  InputPortWidth=3  IndexOptions=Index vector (dialog)  Indices=1  OutputSizes=1
  Conn1 : PMIOPort  Side=Left
  Conn2 : PMIOPort  Port=2  Side=Right
  tag scope: ia=global
  wires:
  Selector/1 -> [ia]
  PS-Simulink Converter/1 -> Selector/1
  connections:
  PS-Simulink Converter/LConn1 -- Current Sensor/RConn1
  Current Sensor/RConn2 -- Conn2/RConn1
  Conn1/RConn1 -- Current Sensor/LConn1

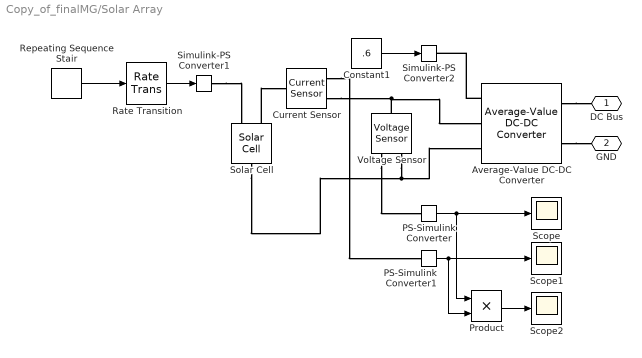
== system Copy_of_finalMG/Solar Array ==
  Average-Value DC-DC Converter : ee_lib/Semiconductors & Converters/Converters/Average-Value DC-DC Converter  implementation_option=ee.enum.converters.implementation.behavioral  converter_type=ee.enum.converters.dcdctype.boost  control_option=ee.enum.converters.controlinput.dutycycle  efficiency_option=ee.enum.converters.efficiency.constant  efficiency_fixed=98  i_vec=[0, 2, 5] A  efficiency_vec=[90, 95, 98]  Lf=1e-6 H  Rl=0 Ohm  Cf=1e-7 F  Rc=1e-6 Ohm  iL_specify=off  iL_priority=High  iL=0 A  iL_nominal_specify=off  iL_nominal_value=1  iL_nominal_unit=A  vc_specify=off  vc_priority=High  vc=0 V  vc_nominal_specify=off  vc_nominal_value=1  vc_nominal_unit=V
      settings: InternalSimscapePortConfiguration="{\"Bottom\":[],\"Left\":[{\"id\":\"DutyCycle\",\"label\":\"DutyCycle\",\"type\":\"input\"},{\"id\":\"p1\",\"label\":\"1+\",\"type\":\"foundation.electrical.electrical\"},{\"id\":\"n1\",\"label\":\"1-\",\"type\":\"foundation.electrical.electrical\"}],\"Right\":[{\"id\":\"p2\",\"label\":\"2+\",\"type\":\"foundation.electrical.electrical\"},{\"id\":\"n2\",\"label\":\"2-\",\"type\":\"foundation.electrical.electrical\"}],\"Top\":[]}"
  Constant1 : Constant  Value=.6
  Current Sensor : fl_lib/Electrical/Electrical Sensors/Current Sensor
  PS-Simulink Converter : nesl_utility/PS-Simulink Converter  PhysicalDomain=network_engine_domain  SubClassName=ps_output  LeftPortType=input  RightPortType=output  PseudoPeriodic=off  Frequencies=[]  VectorFormat=inherit  Unit=inherit  AffineConversion=off
  PS-Simulink Converter1 : nesl_utility/PS-Simulink Converter  PhysicalDomain=network_engine_domain  SubClassName=ps_output  LeftPortType=input  RightPortType=output  PseudoPeriodic=off  Frequencies=[]  VectorFormat=inherit  Unit=inherit  AffineConversion=off
  Product : Product
  Rate Transition : RateTransition
  Repeating Sequence Stair : simulink/Sources/Repeating Sequence Stair  OutValues=irradiance  tsamp=.001  OutMin=[]  OutMax=[]  OutDataTypeStr=double  OutputDataTypeScalingMode=double  OutDataType=fixdt(0,8)  ConRadixGroup=Best Precision: Vector-wise  OutScaling=2^-12
  Scope : Scope
      settings: ActiveDisplayYMinimum=-18.108246963711366  ActiveDisplayYMaximum=460.23470363490452
  Scope1 : Scope
      settings: ActiveDisplayYMinimum=-1  ActiveDisplayYMaximum=1
  Scope2 : Scope
      settings: ActiveDisplayYMinimum=-1  ActiveDisplayYMaximum=1  DataLoggingVariableName=ScopeData2
  Simulink-PS Converter1 : nesl_utility/Simulink-PS Converter  PhysicalDomain=network_engine_domain  SubClassName=ps_input  LeftPortType=input  RightPortType=output  PseudoPeriodic=off  Frequencies=[]  NoiseDistribution=none  NoiseParameters=[]  Unit=1  AffineConversion=off  FilteringAndDerivatives=provide  SimscapeFilterOrder=1  InputFilterTimeConstant=0.001  UdotUserProvided=0
  Simulink-PS Converter2 : nesl_utility/Simulink-PS Converter  PhysicalDomain=network_engine_domain  SubClassName=ps_input  LeftPortType=input  RightPortType=output  PseudoPeriodic=off  Frequencies=[]  NoiseDistribution=none  NoiseParameters=[]  Unit=1  AffineConversion=off  FilteringAndDerivatives=provide  SimscapeFilterOrder=1  InputFilterTimeConstant=0.001  UdotUserProvided=0
  Solar Cell : ee_lib/Sources/Solar Cell  prm=1  Isc=7.34 A  Voc=0.6 V  Is=1e-6 A  Is2=0 A  Iph=7.34 A  Ir0=1000 W/m^2  ec=1.5  N2=2  Rs=0 Ohm  Rp=inf Ohm  N_series=400  N_parallel=20  TIPH1=0 1/K  EG=1.11 eV  TXIS1=3  TXIS2=3  TRS1=0  TRP1=0  Tmeas=25 degC  TFIXED=25 degC  thermal_mass=100 J/K  initial_temperature=25 degC
  Voltage Sensor : fl_lib/Electrical/Electrical Sensors/Voltage Sensor
  DC Bus : PMIOPort  Side=Right
  GND : PMIOPort  Port=2  Side=Right
  wires:
  PS-Simulink Converter/1 -> Product/1, Scope/1
  Constant1/1 -> Simulink-PS Converter2/1
  PS-Simulink Converter1/1 -> Scope1/1, Product/2
  Product/1 -> Scope2/1
  Repeating Sequence Stair/1 -> Rate Transition/1
  Rate Transition/1 -> Simulink-PS Converter1/1
  connections:
  Simulink-PS Converter1/RConn1 -- Solar Cell/LConn1
  Average-Value DC-DC Converter/RConn2 -- GND/RConn1
  Solar Cell/RConn1 -- Voltage Sensor/RConn2 -- Average-Value DC-DC Converter/LConn3
  Average-Value DC-DC Converter/RConn1 -- DC Bus/RConn1
  Voltage Sensor/LConn1 -- Average-Value DC-DC Converter/LConn2 -- Current Sensor/RConn2
  Voltage Sensor/RConn1 -- PS-Simulink Converter/LConn1
  Average-Value DC-DC Converter/LConn1 -- Simulink-PS Converter2/RConn1
  Solar Cell/LConn2 -- Current Sensor/LConn1
  Current Sensor/RConn1 -- PS-Simulink Converter1/LConn1

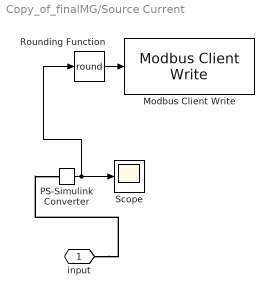
== system Copy_of_finalMG/Source Current ==
  Modbus Client Write : modbuslib/Modbus Client Write  RetainClient=ModbusClient  ClientList=ModbusClient  ConnectionEndpoint=localhost:502  ServerId=1  RegisterTable={ '1', 'Source I', '1', 'Holding Register', 'uint16' }  SampleTime=0.01
  PS-Simulink Converter : nesl_utility/PS-Simulink Converter  PhysicalDomain=network_engine_domain  SubClassName=ps_output  LeftPortType=input  RightPortType=output  PseudoPeriodic=off  Frequencies=[]  VectorFormat=inherit  Unit=inherit  AffineConversion=off
  Rounding Function : Rounding  Operator=round
  Scope : Scope
      settings: ActiveDisplayYMinimum=-0.67540279917219881  ActiveDisplayYMaximum=5.4880807416316095
  input : PMIOPort  Side=Left
  wires:
  PS-Simulink Converter/1 -> Rounding Function/1, Scope/1
  Rounding Function/1 -> Modbus Client Write/1
  connections:
  input/RConn1 -- PS-Simulink Converter/LConn1

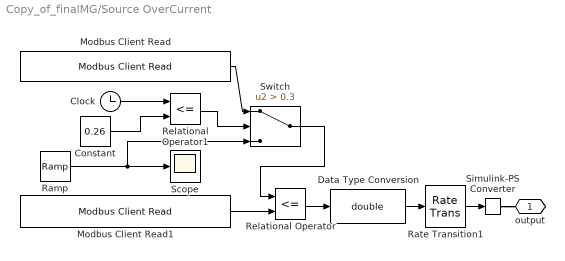
== system Copy_of_finalMG/Source OverCurrent ==
  Clock : Clock
      settings: Decimation=2
  Constant : Constant  Value=0.26
  Data Type Conversion : DataTypeConversion  OutDataTypeStr=double  SaturateOnIntegerOverflow=off  RndMeth=Floor
  Modbus Client Read : modbuslib/Modbus Client Read  RetainClient=ModbusClient  ClientList=ModbusClient  ConnectionEndpoint=localhost:502  ServerId=1  RegisterTable={ '1', 'Source Current', '1', 'Holding Register', 'uint16', '1' }  SampleTime=0.01
  Modbus Client Read1 : modbuslib/Modbus Client Read  RetainClient=ModbusClient  ClientList=ModbusClient  ConnectionEndpoint=localhost:502  ServerId=1  RegisterTable={ '1', 'Limit Current', '3', 'Holding Register', 'uint16', '1' }  SampleTime=0.01
  Ramp : simulink/Sources/Ramp  slope=150  start=0.26  InitialOutput=2
  Rate Transition1 : RateTransition
  Relational Operator : RelationalOperator  Operator=<=  OutDataTypeStr=boolean  RndMeth=Simplest  InputSameDT=off
  Relational Operator1 : RelationalOperator  Operator=<=  OutDataTypeStr=boolean  RndMeth=Simplest  InputSameDT=off
  Scope : Scope
      settings: ActiveDisplayYMinimum=0.76174999999999948  ActiveDisplayYMaximum=13.144250000000007  DataLoggingVariableName=ScopeData5
  Simulink-PS Converter : nesl_utility/Simulink-PS Converter  PhysicalDomain=network_engine_domain  SubClassName=ps_input  LeftPortType=input  RightPortType=output  PseudoPeriodic=off  Frequencies=[]  NoiseDistribution=none  NoiseParameters=[]  Unit=1  AffineConversion=off  FilteringAndDerivatives=provide  SimscapeFilterOrder=1  InputFilterTimeConstant=0.001  UdotUserProvided=0
  Switch : Switch  Criteria=u2 > Threshold  Threshold=0.3  SaturateOnIntegerOverflow=off  InputSameDT=off
  output : PMIOPort  Side=Right
  wires:
  Data Type Conversion/1 -> Rate Transition1/1
  Rate Transition1/1 -> Simulink-PS Converter/1
  Clock/1 -> Relational Operator1/1
  Relational Operator/1 -> Data Type Conversion/1
  Modbus Client Read1/1 -> Relational Operator/2
  Constant/1 -> Relational Operator1/2
  Relational Operator1/1 -> Switch/2
  Modbus Client Read/1 -> Switch/1
  Ramp/1 -> Switch/3, Scope/1
  Switch/1 -> Relational Operator/1
  connections:
  Simulink-PS Converter/RConn1 -- output/RConn1

== system Copy_of_finalMG/Source Voltage ==
  Modbus Client Write1 : modbuslib/Modbus Client Write  RetainClient=ModbusClient  ClientList=ModbusClient  ConnectionEndpoint=localhost:502  ServerId=1  RegisterTable={ '1', 'Source V', '2', 'Holding Register', 'uint16' }  SampleTime=0.01
  Rounding Function1 : Rounding  Operator=round
  Scope2 : Scope
      settings: ActiveDisplayYMinimum=-74.1966496476773  ActiveDisplayYMaximum=667.76984682909585  DataLoggingVariableName=ScopeData2
  wires:
  Rounding Function1/1 -> Modbus Client Write1/1
  [DC_BUS] -> Rounding Function1/1, Scope2/1

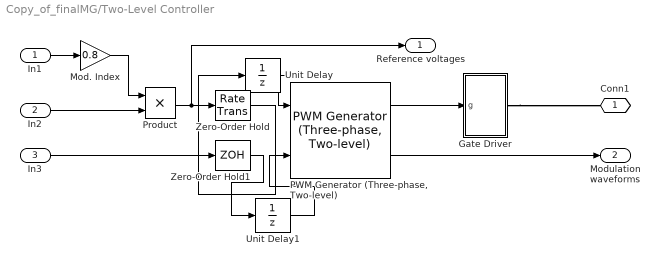
== system Copy_of_finalMG/Two-Level Controller ==
  In1 : Inport
  In2 : Inport  Port=2
  In3 : Inport  Port=3
  Gate Driver : Subsystem
  Mod. Index : Gain  Gain=0.8
  "PWM Generator (Three-phase, Two-level)" : eePwmGeneratorTwoLevel/PWM Generator (Three-phase, Two-level)  PWMMode=Continuous PWM (CPWM)  CPWMMode=SPWM: sinusoidal PWM  DPWMMode=60 DPWM: 60 degree discontinuous PWM  fsw=1e3  Ts=Ts
  Product : Product
  Unit Delay : UnitDelay  SampleTime=-1  HasFrameUpgradeWarning=on
  Unit Delay1 : UnitDelay  SampleTime=-1  HasFrameUpgradeWarning=on
  Zero-Order Hold : RateTransition  OutPortSampleTime=0.0001
  Zero-Order Hold1 : ZeroOrderHold  SampleTime=0.0001
  Conn1 : PMIOPort  Side=Right
  Reference voltages : Outport  VectorParamsAs1DForOutWhenUnconnected=off
  Modulation waveforms : Outport  Port=2  VectorParamsAs1DForOutWhenUnconnected=off
  wires:
  Product/1 -> Reference voltages/1, Zero-Order Hold/1
  Zero-Order Hold1/1 -> Unit Delay1/1
  Zero-Order Hold/1 -> Unit Delay/1
  In2/1 -> Product/2
  In3/1 -> Zero-Order Hold1/1
  "PWM Generator (Three-phase, Two-level)"/1 -> Gate Driver/1(g)
  "PWM Generator (Three-phase, Two-level)"/2 -> Modulation waveforms/1
  Mod. Index/1 -> Product/1
  In1/1 -> Mod. Index/1
  Unit Delay/1 -> "PWM Generator (Three-phase, Two-level)"/1
  Unit Delay1/1 -> "PWM Generator (Three-phase, Two-level)"/2
  connections:
  Gate Driver/RConn1 -- Conn1/RConn1

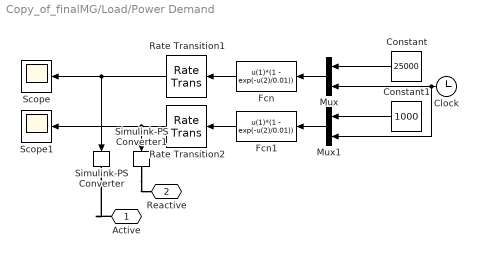
== system Copy_of_finalMG/Load/Power Demand ==
  Clock : Clock
  Constant : Constant  Value=25000
  Constant1 : Constant  Value=1000
  Fcn : Fcn  Expr=u(1)*(1 - exp(-u(2)/0.01))
  Fcn1 : Fcn  Expr=u(1)*(1 - exp(-u(2)/0.01))
  Mux : Mux  Inputs=2
  Mux1 : Mux  Inputs=2
  Rate Transition1 : RateTransition
  Rate Transition2 : RateTransition
  Scope : Scope
      settings: ActiveDisplayYMinimum=-1  ActiveDisplayYMaximum=1  DataLoggingVariableName=ScopeData6
  Scope1 : Scope
      settings: DataLoggingVariableName=ScopeData9
  Simulink-PS Converter : nesl_utility/Simulink-PS Converter  PhysicalDomain=network_engine_domain  SubClassName=ps_input  LeftPortType=input  RightPortType=output  PseudoPeriodic=off  Frequencies=[]  NoiseDistribution=none  NoiseParameters=[]  Unit=1  AffineConversion=off  FilteringAndDerivatives=provide  SimscapeFilterOrder=1  InputFilterTimeConstant=0.001  UdotUserProvided=0
  Simulink-PS Converter1 : nesl_utility/Simulink-PS Converter  PhysicalDomain=network_engine_domain  SubClassName=ps_input  LeftPortType=input  RightPortType=output  PseudoPeriodic=off  Frequencies=[]  NoiseDistribution=none  NoiseParameters=[]  Unit=1  AffineConversion=off  FilteringAndDerivatives=provide  SimscapeFilterOrder=1  InputFilterTimeConstant=0.001  UdotUserProvided=0
  Active : PMIOPort  Side=Left
  Reactive : PMIOPort  Port=2  Side=Left
  wires:
  Constant1/1 -> Mux1/1
  Fcn1/1 -> Rate Transition2/1
  Fcn/1 -> Rate Transition1/1
  Constant/1 -> Mux/1
  Clock/1 -> Mux1/2, Mux/2
  Rate Transition2/1 -> Scope1/1, Simulink-PS Converter1/1
  Mux1/1 -> Fcn1/1
  Rate Transition1/1 -> Scope/1, Simulink-PS Converter/1
  Mux/1 -> Fcn/1
  connections:
  Simulink-PS Converter1/RConn1 -- Reactive/RConn1
  Active/RConn1 -- Simulink-PS Converter/RConn1

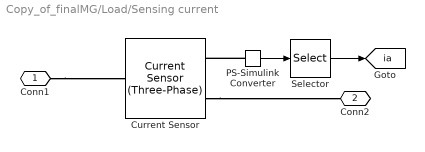
== system Copy_of_finalMG/Load/Sensing current ==
  Current Sensor : ee_lib/Sensors & Transducers/Current Sensor (Three-Phase)
  PS-Simulink Converter : nesl_utility/PS-Simulink Converter  PhysicalDomain=network_engine_domain  SubClassName=ps_output  LeftPortType=input  RightPortType=output  PseudoPeriodic=off  Frequencies=[]  VectorFormat=1-D array  Unit=1  AffineConversion=off
  Selector : Selector  InputPortWidth=3  IndexOptions=Index vector (dialog)  Indices=1  OutputSizes=1
  Conn1 : PMIOPort  Side=Left
  Conn2 : PMIOPort  Port=2  Side=Right
  tag scope: ia=global
  wires:
  Selector/1 -> [ia]
  PS-Simulink Converter/1 -> Selector/1
  connections:
  PS-Simulink Converter/LConn1 -- Current Sensor/RConn1
  Current Sensor/RConn2 -- Conn2/RConn1
  Conn1/RConn1 -- Current Sensor/LConn1

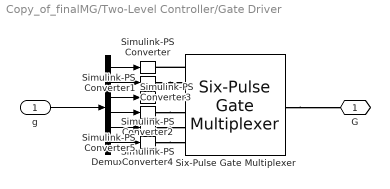
== system Copy_of_finalMG/Two-Level Controller/Gate Driver ==
  g : Inport
  Demux : Demux  Outputs=6
  Simulink-PS Converter{,1..5} (6 alike) : nesl_utility/Simulink-PS Converter  PhysicalDomain=network_engine_domain  SubClassName=ps_input  LeftPortType=input  RightPortType=output  PseudoPeriodic=off  Frequencies=[]  NoiseDistribution=none  NoiseParameters=[]  Unit=1  AffineConversion=off  FilteringAndDerivatives=zero  SimscapeFilterOrder=1  InputFilterTimeConstant=0.001  UdotUserProvided=1
  Six-Pulse Gate Multiplexer : ee_lib/Semiconductors & Converters/Converters/Six-Pulse Gate Multiplexer  port_option=ee.enum.controlport.ps
  G : PMIOPort  Side=Right
  wires:
  g/1 -> Demux/1
  Demux/1 -> Simulink-PS Converter/1
  Demux/2 -> Simulink-PS Converter1/1
  Demux/3 -> Simulink-PS Converter2/1
  Demux/4 -> Simulink-PS Converter3/1
  Demux/5 -> Simulink-PS Converter4/1
  Demux/6 -> Simulink-PS Converter5/1
  connections:
  Six-Pulse Gate Multiplexer/LConn1 -- Simulink-PS Converter/RConn1
  Simulink-PS Converter1/RConn1 -- Six-Pulse Gate Multiplexer/LConn2
  Simulink-PS Converter2/RConn1 -- Six-Pulse Gate Multiplexer/LConn3
  Simulink-PS Converter3/RConn1 -- Six-Pulse Gate Multiplexer/LConn4
  Simulink-PS Converter4/RConn1 -- Six-Pulse Gate Multiplexer/LConn5
  Simulink-PS Converter5/RConn1 -- Six-Pulse Gate Multiplexer/LConn6
  Six-Pulse Gate Multiplexer/RConn1 -- G/RConn1
